simulink model "SWC_FDC_type"  (R2021b)
settings: Solver=FixedStepDiscrete  StartTime=0.0  StopTime=10.0  FixedStep=0.001  RelTol=1e-3
values from neighbouring files (symbols this model uses):
  C_TASK_5MS_S = (	C_TICK_TIME_S      	)    [vcu_local_hdr.m]
  DID_VCUKey = uint16(0x0202)    [vcu_local_hdr.m]
  DID_XWD = uint16(513)    [vcu_local_hdr.m]
  DIDLen_DKCKey = uint16(8)    [vcu_local_hdr.m]
  DIDLen_FoxPiBattSta = uint16(4)    [vcu_local_hdr.m]
  DIDLen_FoxPiBrakeSta = uint16(13)    [vcu_local_hdr.m]
  DIDLen_FoxPiButtonSta = uint16(2)    [vcu_local_hdr.m]
  DIDLen_FoxPiCtrlEnSw = uint16(1)    [vcu_local_hdr.m]
  DIDLen_FoxPiDrivingCtrl = uint16(21)    [vcu_local_hdr.m]
  DIDLen_FoxPiEPSSta = uint16(11)    [vcu_local_hdr.m]
  DIDLen_FoxPiLampCtrl = uint16(6)    [vcu_local_hdr.m]
  DIDLen_FoxPiLampSta = uint16(2)    [vcu_local_hdr.m]
  DIDLen_FoxPiMotionSta = uint16(13)    [vcu_local_hdr.m]
  DIDLen_FoxPiMotorSta = uint16(11)    [vcu_local_hdr.m]
  DIDLen_FoxPiPedalPos = uint16(3)    [vcu_local_hdr.m]
  DIDLen_FoxPiPTGUSSSw = uint16(1)    [vcu_local_hdr.m]
  DIDLen_FoxPiShifterAllow = uint16(3)    [vcu_local_hdr.m]
  DIDLen_FoxPiSwSta = uint16(2)    [vcu_local_hdr.m]
  DIDLen_FoxPiTPMSSta = uint16(13)    [vcu_local_hdr.m]
  DIDLen_FoxPiUSSDist = uint16(20)    [vcu_local_hdr.m]
  DIDLen_FoxPiUSSFaultSta = uint16(2)    [vcu_local_hdr.m]
  DIDLen_FoxPiWheelSpd = uint16(16)    [vcu_local_hdr.m]
  DIDNum_DKCKey = uint16(0x0202)    [vcu_local_hdr.m]
  DIDNum_FoxPiBattSta = uint16(0x100D)    [vcu_local_hdr.m]
  DIDNum_FoxPiBrakeSta = uint16(0x1003)    [vcu_local_hdr.m]
  DIDNum_FoxPiButtonSta = uint16(0x1006)    [vcu_local_hdr.m]
  DIDNum_FoxPiCtrlEnSw = uint16(0x1012)    [vcu_local_hdr.m]
  DIDNum_FoxPiDrivingCtrl = uint16(0x1001)    [vcu_local_hdr.m]
  DIDNum_FoxPiEPSSta = uint16(0x1005)    [vcu_local_hdr.m]
  DIDNum_FoxPiLampCtrl = uint16(0x100C)    [vcu_local_hdr.m]
  DIDNum_FoxPiLampSta = uint16(0x100B)    [vcu_local_hdr.m]
  DIDNum_FoxPiMotionSta = uint16(0x1002)    [vcu_local_hdr.m]
  DIDNum_FoxPiMotorSta = uint16(0x1010)    [vcu_local_hdr.m]
  DIDNum_FoxPiPedalPos = uint16(0x100F)    [vcu_local_hdr.m]
  DIDNum_FoxPiPTGUSSSw = uint16(0x1009)    [vcu_local_hdr.m]
  DIDNum_FoxPiShifterAllow = uint16(0x1011)    [vcu_local_hdr.m]
  DIDNum_FoxPiSwSta = uint16(0x100A)    [vcu_local_hdr.m]
  DIDNum_FoxPiTPMSSta = uint16(0x100E)    [vcu_local_hdr.m]
  DIDNum_FoxPiUSSDist = uint16(0x1007)    [vcu_local_hdr.m]
  DIDNum_FoxPiUSSFaultSta = uint16(0x1008)    [vcu_local_hdr.m]
  DIDNum_FoxPiWheelSpd = uint16(0x1004)    [vcu_local_hdr.m]
  DIDVCUKeyLength = uint16(8)    [vcu_local_hdr.m]
  DTC_10020B = Simulink.Parameter    [DTC_Constant_Definition.m]
  DTC_10020C = Simulink.Parameter    [DTC_Constant_Definition.m]
  DTC_10020D = Simulink.Parameter    [DTC_Constant_Definition.m]
  DTC_10020E = Simulink.Parameter    [DTC_Constant_Definition.m]
  DTC_100210 = Simulink.Parameter    [DTC_Constant_Definition.m]
  DTC_100211 = Simulink.Parameter    [DTC_Constant_Definition.m]
  DTC_100212 = Simulink.Parameter    [DTC_Constant_Definition.m]
  DTC_100213 = Simulink.Parameter    [DTC_Constant_Definition.m]
  DTC_100214 = Simulink.Parameter    [DTC_Constant_Definition.m]
  DTC_100215 = Simulink.Parameter    [DTC_Constant_Definition.m]
  DTC_100216 = Simulink.Parameter    [DTC_Constant_Definition.m]
  DTC_100217 = Simulink.Parameter    [DTC_Constant_Definition.m]
  DTC_100218 = Simulink.Parameter    [DTC_Constant_Definition.m]
  DTC_100219 = Simulink.Parameter    [DTC_Constant_Definition.m]
  DTC_10021A = Simulink.Parameter    [DTC_Constant_Definition.m]
  DTC_10021B = Simulink.Parameter    [DTC_Constant_Definition.m]
  DTC_10021C = Simulink.Parameter    [DTC_Constant_Definition.m]
  DTC_10021D = Simulink.Parameter    [DTC_Constant_Definition.m]
  DTC_10021E = Simulink.Parameter    [DTC_Constant_Definition.m]
  DTC_100220 = Simulink.Parameter    [DTC_Constant_Definition.m]
  DTC_100221 = Simulink.Parameter    [DTC_Constant_Definition.m]
  DTC_100223 = Simulink.Parameter    [DTC_Constant_Definition.m]
  DTC_100224 = Simulink.Parameter    [DTC_Constant_Definition.m]
  DTC_100225 = Simulink.Parameter    [DTC_Constant_Definition.m]
  DTC_100226 = Simulink.Parameter    [DTC_Constant_Definition.m]
  DTC_100227 = Simulink.Parameter    [DTC_Constant_Definition.m]
  DTC_100242 = Simulink.Parameter    [DTC_Constant_Definition.m]
  DTC_100243 = Simulink.Parameter    [DTC_Constant_Definition.m]
  DTC_100244 = Simulink.Parameter    [DTC_Constant_Definition.m]
  DTC_100247 = Simulink.Parameter    [DTC_Constant_Definition.m]
  DTC_100248 = Simulink.Parameter    [DTC_Constant_Definition.m]
  DTC_100249 = Simulink.Parameter    [DTC_Constant_Definition.m]
  DTC_100250 = Simulink.Parameter    [DTC_Constant_Definition.m]
  DTC_100251 = Simulink.Parameter    [DTC_Constant_Definition.m]
  DTC_100252 = Simulink.Parameter    [DTC_Constant_Definition.m]
  DTC_100A10 = Simulink.Parameter    [DTC_Constant_Definition.m]
  DTC_100A12 = Simulink.Parameter    [DTC_Constant_Definition.m]
  DTC_100A16 = Simulink.Parameter    [DTC_Constant_Definition.m]
  DTC_100A17 = Simulink.Parameter    [DTC_Constant_Definition.m]
  DTC_100A18 = Simulink.Parameter    [DTC_Constant_Definition.m]
  DTC_100A19 = Simulink.Parameter    [DTC_Constant_Definition.m]
  DTC_500B01 = Simulink.Parameter    [DTC_Constant_Definition.m]
  DTC_500B02 = Simulink.Parameter    [DTC_Constant_Definition.m]
  DTC_500B03 = Simulink.Parameter    [DTC_Constant_Definition.m]
  DTC_500B04 = Simulink.Parameter    [DTC_Constant_Definition.m]
  DTC_500B05 = Simulink.Parameter    [DTC_Constant_Definition.m]
  DTC_500B06 = Simulink.Parameter    [DTC_Constant_Definition.m]
  DTC_500B07 = Simulink.Parameter    [DTC_Constant_Definition.m]
  DTC_500B08 = Simulink.Parameter    [DTC_Constant_Definition.m]
  DTC_500B09 = Simulink.Parameter    [DTC_Constant_Definition.m]
  DTC_500B0A = Simulink.Parameter    [DTC_Constant_Definition.m]
  DTC_500B0B = Simulink.Parameter    [DTC_Constant_Definition.m]
  DTC_500B0C = Simulink.Parameter    [DTC_Constant_Definition.m]
  DTC_500B0D = Simulink.Parameter    [DTC_Constant_Definition.m]
  DTC_500B0E = Simulink.Parameter    [DTC_Constant_Definition.m]
  DTC_500B0F = Simulink.Parameter    [DTC_Constant_Definition.m]
  DTC_500B10 = Simulink.Parameter    [DTC_Constant_Definition.m]
  DTC_90021F = Simulink.Parameter    [DTC_Constant_Definition.m]
  DTC_90022F = Simulink.Parameter    [DTC_Constant_Definition.m]
  DTC_900253 = Simulink.Parameter    [DTC_Constant_Definition.m]
  DTC_900254 = Simulink.Parameter    [DTC_Constant_Definition.m]
  DTC_900301 = Simulink.Parameter    [DTC_Constant_Definition.m]
  DTC_900302 = Simulink.Parameter    [DTC_Constant_Definition.m]
  DTC_900303 = Simulink.Parameter    [DTC_Constant_Definition.m]
  DTC_900304 = Simulink.Parameter    [DTC_Constant_Definition.m]
  DTC_900305 = Simulink.Parameter    [DTC_Constant_Definition.m]
  DTC_900909 = Simulink.Parameter    [DTC_Constant_Definition.m]
  DTC_90090A = Simulink.Parameter    [DTC_Constant_Definition.m]
  DTC_90090B = Simulink.Parameter    [DTC_Constant_Definition.m]
  DTC_90090C = Simulink.Parameter    [DTC_Constant_Definition.m]
  DTC_90090D = Simulink.Parameter    [DTC_Constant_Definition.m]
  DTC_90090E = Simulink.Parameter    [DTC_Constant_Definition.m]
  DTC_90090F = Simulink.Parameter    [DTC_Constant_Definition.m]
  DTC_900910 = Simulink.Parameter    [DTC_Constant_Definition.m]
  DTC_900911 = Simulink.Parameter    [DTC_Constant_Definition.m]
  DTC_900912 = Simulink.Parameter    [DTC_Constant_Definition.m]
  DTC_900913 = Simulink.Parameter    [DTC_Constant_Definition.m]
  DTC_900914 = Simulink.Parameter    [DTC_Constant_Definition.m]
  ... (+54 more)
undefined symbols (not defined in the file or in its folder): f32_ApsOutVehSpdSig, KHAL_CANBusOffDebounce_cnt, KHAL_CANBusOffDebounce_s, KHAL_DKCDecryptEnable_flg_ovrdflg, KHAL_DKCDecryptEnable_flg_ovrdval, KHAL_RandomNumberY1_enum, KHAL_RandomNumberY2_enum, KHAL_RandomNumberY_ovrdflg, KHAL_TPMSRESBUTT_flg_ovrdflg, KHAL_TPMSRESBUTT_flg_ovrdval, KINP_ReadVinCode_flg, P_boolean, R_DIDWriteCDD_CSOP_DIDSet_DKCKey, R_DIDWriteCDD_CSOP_DIDSet_FoxPiBattSta, R_DIDWriteCDD_CSOP_DIDSet_FoxPiBrakeSta, R_DIDWriteCDD_CSOP_DIDSet_FoxPiButtonSta, R_DIDWriteCDD_CSOP_DIDSet_FoxPiCtrlEnSw, R_DIDWriteCDD_CSOP_DIDSet_FoxPiDrivingCtrl, R_DIDWriteCDD_CSOP_DIDSet_FoxPiEPSSta, R_DIDWriteCDD_CSOP_DIDSet_FoxPiLampCtrl, R_DIDWriteCDD_CSOP_DIDSet_FoxPiLampSta, R_DIDWriteCDD_CSOP_DIDSet_FoxPiMotionSta, R_DIDWriteCDD_CSOP_DIDSet_FoxPiMotorSta, R_DIDWriteCDD_CSOP_DIDSet_FoxPiPedalPos, R_DIDWriteCDD_CSOP_DIDSet_FoxPiPTGUSSSw, R_DIDWriteCDD_CSOP_DIDSet_FoxPiShifterAllow, R_DIDWriteCDD_CSOP_DIDSet_FoxPiSwSta, R_DIDWriteCDD_CSOP_DIDSet_FoxPiTPMSSta, R_DIDWriteCDD_CSOP_DIDSet_FoxPiUSSDist, R_DIDWriteCDD_CSOP_DIDSet_FoxPiUSSFaultSta, R_DIDWriteCDD_CSOP_DIDSet_FoxPiWheelSpd, R_E2E_CAN3_VCU1_CSOP_Write_CAN3_VCU1, R_E2E_CAN3_VCU1_toNIDEC_CSOP_Write_CAN3_VCU1_toNIDEC, R_E2E_CAN4_VCU1_CSOP_Write_CAN4_VCU1, R_FDCCDD_Inner_CSOP_FDC_AppCallSleep, R_HALIN_IMU_CSOP_IMUSetSta, R_HALINCDD_CSOP_PAS_Handler, R_HALINCDD_CSOP_ResetPedalZeroPosDone, R_HALINCDD_CSOP_TPMSSensorIDRegSetResults, R_HALINCDD_CSOP_UDS_Main, R_HALOUT_APS_CSOP_ApsOutput, R_HALOUTCDD_CSOP_AppNmStateReq, R_HALOUTCDD_CSOP_IVIReset, R_HALOUTCDD_CSOP_SetAcoreRebootCmdACK, R_HALOUTCDD_CSOP_SetSysPwrStat ... (+80)
libraries: FVT_lib x447, simulink x289, hcu_lib x19, hdlsllib x9, app x1, halin x1, halout x1, matrix_library x1, inp x1, outp x1
(part 8 of 15)

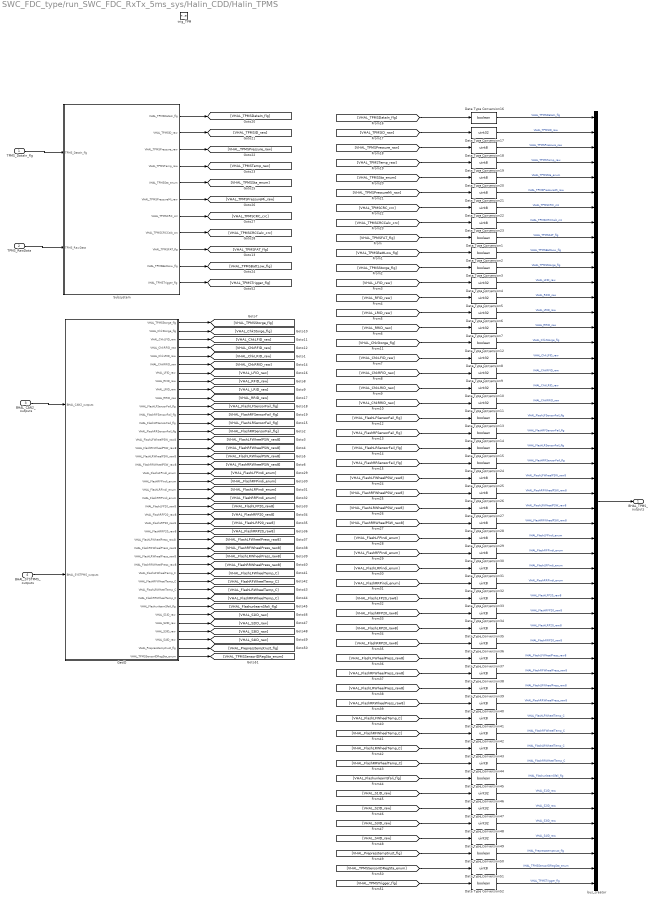
== system SWC_FDC_type/run_SWC_FDC_RxTx_5ms_sys/Halin_CDD/Halin_TPMS ==
  TPMS_DataIn_flg : Inport
  TPMS_RawData : Inport  Port=2
  BHAL_CAN2_outputs : Inport  Port=3
  BHAL_SYSTPMS_outputs : Inport  Port=4
  trig_TPM : TriggerPort  TriggerType=function-call  VariantControl=(inherit)
  Data Type Conversion{1..3,12..16,24,45,50,52} (12 alike) : DataTypeConversion  OutDataTypeStr=boolean
  Data Type Conversion{4..11,17,46..49} (13 alike) : DataTypeConversion  OutDataTypeStr=uint32
  Data Type Conversion{18..23,25..44,51} (27 alike) : DataTypeConversion  OutDataTypeStr=uint8
  GetID : Subsystem
  Subsystem : Subsystem
  bus_creator : BusCreator  Inputs=52  OutDataTypeStr=Bus: BHAL_TPMS_outputs  NonVirtualBus=on
  BHAL_TPMS_outputs : Outport
  wires:
  Subsystem/8(VHAL_TPMSCRCCalc_crc) -> [VHAL_TPMSCRCCalc_crc]
  Subsystem/7(VHAL_TPMSCRC_crc) -> [VHAL_TPMSCRC_crc]
  Subsystem/1(VHAL_TPMSDataIn_flg) -> [VHAL_TPMSDataIn_flg]
  Subsystem/9(VHAL_TPMSFAT_flg) -> [VHAL_TPMSFAT_flg]
  Subsystem/2(VHAL_TPMSID_raw) -> [VHAL_TPMSID_raw]
  Subsystem/10(VHAL_TPMSBattLow_flg) -> [VHAL_TPMSBattLow_flg]
  Subsystem/4(VHAL_TPMSTemp_raw) -> [VHAL_TPMSTemp_raw]
  Subsystem/5(VHAL_TPMSSta_enum) -> [VHAL_TPMSSta_enum]
  Subsystem/3(VHAL_TPMSPressure_raw) -> [VHAL_TPMSPressure_raw]
  Subsystem/6(VHAL_TPMSPressureMi_raw) -> [VHAL_TPMSPressureMi_raw]
  TPMS_DataIn_flg/1 -> Subsystem/1(TPMS_DataIn_flg)
  TPMS_RawData/1 -> Subsystem/2(TPMS_RawData)
  Data Type Conversion29/1 -> bus_creator/29  "VHAL_FlashLFPindi_enum"
  GetID/20(VHAL_FlashRFPindi_enum) -> [VHAL_FlashRFPindi_enum]
  GetID/32(VHAL_FlashRFWheelTemp_C) -> [VHAL_FlashRFWheelTemp_C]
  Data Type Conversion2/1 -> bus_creator/10  "VHAL_TPMSBattLow_flg"
  BHAL_CAN2_outputs/1 -> GetID/1(BHAL_CAN2_outputs)
  [VHAL_TPMSBattLow_flg] -> Data Type Conversion2/1
  [VHAL_FlashLRPindi_enum] -> Data Type Conversion31/1
  [VHAL_FlashunlearnSfali_flg] -> Data Type Conversion45/1
  [VHAL_FlashLFPindi_enum] -> Data Type Conversion29/1
  Data Type Conversion28/1 -> bus_creator/28  "VHAL_FlashRRWheelPSW_raw8"
  [VHAL_FlashLFP20_raw8] -> Data Type Conversion33/1
  [VHAL_RRID_raw] -> Data Type Conversion7/1
  Data Type Conversion42/1 -> bus_creator/42  "VHAL_FlashRFWheelTemp_C"
  Data Type Conversion27/1 -> bus_creator/27  "VHAL_FlashLRWheelPSW_raw8"
  [VHAL_FlashLFWheelTemp_C] -> Data Type Conversion41/1
  Data Type Conversion26/1 -> bus_creator/26  "VHAL_FlashRFWheelPSW_raw8"
  [VHAL_FlashRRP20_raw8] -> Data Type Conversion36/1
  GetID/16(VHAL_FlashRFWheelPSW_raw8) -> [VHAL_FlashRFWheelPSW_raw8]
  [VHAL_RFID_raw] -> Data Type Conversion5/1
  Data Type Conversion33/1 -> bus_creator/33  "VHAL_FlashLFP20_raw8"
  Data Type Conversion24/1 -> bus_creator/24  "VHAL_FlashRRSensorFail_flg"
  Data Type Conversion44/1 -> bus_creator/44  "VHAL_FlashRRWheelTemp_C"
  Data Type Conversion34/1 -> bus_creator/34  "VHAL_FlashRFP20_raw8"
  Data Type Conversion45/1 -> bus_creator/45  "VHAL_FlashunlearnSfali_flg"
  GetID/9(VHAL_LRID_raw) -> [VHAL_LRID_raw]
  Data Type Conversion41/1 -> bus_creator/41  "VHAL_FlashLFWheelTemp_C"
  GetID/15(VHAL_FlashLFWheelPSW_raw8) -> [VHAL_FlashLFWheelPSW_raw8]
  Data Type Conversion15/1 -> bus_creator/23  "VHAL_FlashLRSensorFail_flg"
  [VHAL_FlashLRWheelPress_raw8] -> Data Type Conversion39/1
  Data Type Conversion14/1 -> bus_creator/22  "VHAL_FlashRFSensorFail_flg"
  GetID/34(VHAL_FlashRRWheelTemp_C) -> [VHAL_FlashRRWheelTemp_C]
  Data Type Conversion13/1 -> bus_creator/21  "VHAL_FlashLFSensorFail_flg"
  Data Type Conversion32/1 -> bus_creator/32  "VHAL_FlashRRPindi_enum"
  Data Type Conversion31/1 -> bus_creator/31  "VHAL_FlashLRPindi_enum"
  Data Type Conversion16/1 -> bus_creator/1  "VHAL_TPMSDataIn_flg"
  GetID/22(VHAL_FlashRRPindi_enum) -> [VHAL_FlashRRPindi_enum]
  [VHAL_FlashRFSensorFail_flg] -> Data Type Conversion14/1
  GetID/18(VHAL_FlashRRWheelPSW_raw8) -> [VHAL_FlashRRWheelPSW_raw8]
  Data Type Conversion43/1 -> bus_creator/43  "VHAL_FlashLRWheelTemp_C"
  Data Type Conversion22/1 -> bus_creator/7  "VHAL_TPMSCRC_crc"
  Data Type Conversion40/1 -> bus_creator/40  "VHAL_FlashRRWheelPress_raw8"
  Data Type Conversion39/1 -> bus_creator/39  "VHAL_FlashLRWheelPress_raw8"
  [VHAL_FlashRRPindi_enum] -> Data Type Conversion32/1
  Data Type Conversion38/1 -> bus_creator/38  "VHAL_FlashRFWheelPress_raw8"
  [VHAL_FlashLRP20_raw8] -> Data Type Conversion35/1
  Data Type Conversion35/1 -> bus_creator/35  "VHAL_FlashLRP20_raw8"
  GetID/14(VHAL_FlashRRSensorFail_flg) -> [VHAL_FlashRRSensorFail_flg]
  Data Type Conversion37/1 -> bus_creator/37  "VHAL_FlashLFWheelPress_raw8"
  Data Type Conversion36/1 -> bus_creator/36  "VHAL_FlashRRP20_raw8"
  [VHAL_FlashRRWheelTemp_C] -> Data Type Conversion44/1
  [VHAL_FlashLFWheelPress_raw8] -> Data Type Conversion37/1
  GetID/33(VHAL_FlashLRWheelTemp_C) -> [VHAL_FlashLRWheelTemp_C]
  GetID/26(VHAL_FlashRRP20_raw8) -> [VHAL_FlashRRP20_raw8]
  [VHAL_TPMSFAT_flg] -> Data Type Conversion1/1
  [VHAL_TPMSSta_enum] -> Data Type Conversion20/1
  GetID/25(VHAL_FlashLRP20_raw8) -> [VHAL_FlashLRP20_raw8]
  [VHAL_FlashRRWheelPress_raw8] -> Data Type Conversion40/1
  [VHAL_FlashRFP20_raw8] -> Data Type Conversion34/1
  [VHAL_LFID_raw] -> Data Type Conversion4/1
  [VHAL_FlashRFWheelPSW_raw8] -> Data Type Conversion26/1
  [VHAL_FlashRFWheelTemp_C] -> Data Type Conversion42/1
  [VHAL_FlashLRWheelTemp_C] -> Data Type Conversion43/1
  [VHAL_TPMSCRCCalc_crc] -> Data Type Conversion23/1
  GetID/31(VHAL_FlashLFWheelTemp_C) -> [VHAL_FlashLFWheelTemp_C]
  [VHAL_FlashRRSensorFail_flg] -> Data Type Conversion24/1
  [VHAL_FlashLFSensorFail_flg] -> Data Type Conversion13/1
  GetID/30(VHAL_FlashRRWheelPress_raw8) -> [VHAL_FlashRRWheelPress_raw8]
  Data Type Conversion3/1 -> bus_creator/11  "VHAL_TPMSStorge_flg"
  GetID/29(VHAL_FlashLRWheelPress_raw8) -> [VHAL_FlashLRWheelPress_raw8]
  GetID/21(VHAL_FlashLRPindi_enum) -> [VHAL_FlashLRPindi_enum]
  GetID/1(VHAL_TPMSStorge_flg) -> [VHAL_TPMSStorge_flg]
  [VHAL_FlashRFPindi_enum] -> Data Type Conversion30/1
  GetID/19(VHAL_FlashLFPindi_enum) -> [VHAL_FlashLFPindi_enum]
  GetID/23(VHAL_FlashLFP20_raw8) -> [VHAL_FlashLFP20_raw8]
  Data Type Conversion6/1 -> bus_creator/14  "VHAL_LRID_raw"
  GetID/6(VHAL_ChkRRID_raw) -> [VHAL_ChkRRID_raw]
  [VHAL_TPMSDataIn_flg] -> Data Type Conversion16/1
  GetID/17(VHAL_FlashLRWheelPSW_raw8) -> [VHAL_FlashLRWheelPSW_raw8]
  [VHAL_FlashRFWheelPress_raw8] -> Data Type Conversion38/1
  Data Type Conversion1/1 -> bus_creator/9  "VHAL_TPMSFAT_flg"
  GetID/3(VHAL_ChkLFID_raw) -> [VHAL_ChkLFID_raw]
  GetID/35(VHAL_FlashunlearnSfali_flg) -> [VHAL_FlashunlearnSfali_flg]
  [VHAL_FlashLFWheelPSW_raw8] -> Data Type Conversion25/1
  GetID/8(VHAL_RFID_raw) -> [VHAL_RFID_raw]
  GetID/10(VHAL_RRID_raw) -> [VHAL_RRID_raw]
  Data Type Conversion12/1 -> bus_creator/16  "VHAL_ChkStorge_flg"
  [VHAL_FlashLRWheelPSW_raw8] -> Data Type Conversion27/1
  GetID/7(VHAL_LFID_raw) -> [VHAL_LFID_raw]
  Data Type Conversion18/1 -> bus_creator/3  "VHAL_TPMSPressure_raw"
  Data Type Conversion9/1 -> bus_creator/18  "VHAL_ChkRFID_raw"
  Data Type Conversion10/1 -> bus_creator/19  "VHAL_ChkLRID_raw"
  GetID/11(VHAL_FlashLFSensorFail_flg) -> [VHAL_FlashLFSensorFail_flg]
  GetID/27(VHAL_FlashLFWheelPress_raw8) -> [VHAL_FlashLFWheelPress_raw8]
  Data Type Conversion11/1 -> bus_creator/20  "VHAL_ChkRRID_raw"
  Data Type Conversion7/1 -> bus_creator/15  "VHAL_RRID_raw"
  GetID/4(VHAL_ChkRFID_raw) -> [VHAL_ChkRFID_raw]
  [VHAL_TPMSID_raw] -> Data Type Conversion17/1
  [VHAL_ChkStorge_flg] -> Data Type Conversion12/1
  GetID/28(VHAL_FlashRFWheelPress_raw8) -> [VHAL_FlashRFWheelPress_raw8]
  Data Type Conversion8/1 -> bus_creator/17  "VHAL_ChkLFID_raw"
  [VHAL_ChkRRID_raw] -> Data Type Conversion11/1
  Data Type Conversion4/1 -> bus_creator/12  "VHAL_LFID_raw"
  [VHAL_ChkLRID_raw] -> Data Type Conversion10/1
  [VHAL_ChkLFID_raw] -> Data Type Conversion8/1
  [VHAL_ChkRFID_raw] -> Data Type Conversion9/1
  Data Type Conversion5/1 -> bus_creator/13  "VHAL_RFID_raw"
  [VHAL_LRID_raw] -> Data Type Conversion6/1
  [VHAL_TPMSStorge_flg] -> Data Type Conversion3/1
  GetID/2(VHAL_ChkStorge_flg) -> [VHAL_ChkStorge_flg]
  [VHAL_TPMSCRC_crc] -> Data Type Conversion22/1
  Data Type Conversion19/1 -> bus_creator/4  "VHAL_TPMSTemp_raw"
  BHAL_SYSTPMS_outputs/1 -> GetID/2(BHAL_SYSTPMS_outputs)
  [VHAL_FlashLRSensorFail_flg] -> Data Type Conversion15/1
  Data Type Conversion17/1 -> bus_creator/2  "VHAL_TPMSID_raw"
  Data Type Conversion23/1 -> bus_creator/8  "VHAL_TPMSCRCCalc_crc"
  Data Type Conversion30/1 -> bus_creator/30  "VHAL_FlashRFPindi_enum"
  Data Type Conversion21/1 -> bus_creator/6  "VHAL_TPMSPressureMi_raw"
  GetID/5(VHAL_ChkLRID_raw) -> [VHAL_ChkLRID_raw]
  [VHAL_TPMSTemp_raw] -> Data Type Conversion19/1
  GetID/13(VHAL_FlashLRSensorFail_flg) -> [VHAL_FlashLRSensorFail_flg]
  [VHAL_TPMSPressure_raw] -> Data Type Conversion18/1
  GetID/24(VHAL_FlashRFP20_raw8) -> [VHAL_FlashRFP20_raw8]
  bus_creator/1 -> BHAL_TPMS_outputs/1
  Data Type Conversion20/1 -> bus_creator/5  "VHAL_TPMSSta_enum"
  Data Type Conversion25/1 -> bus_creator/25  "VHAL_FlashLFWheelPSW_raw8"
  [VHAL_TPMSPressureMi_raw] -> Data Type Conversion21/1
  GetID/12(VHAL_FlashRFSensorFail_flg) -> [VHAL_FlashRFSensorFail_flg]
  [VHAL_FlashRRWheelPSW_raw8] -> Data Type Conversion28/1
  GetID/36(VHAL_S1ID_raw) -> [VHAL_S1ID_raw]
  GetID/37(VHAL_S2ID_raw) -> [VHAL_S2ID_raw]
  GetID/38(VHAL_S3ID_raw) -> [VHAL_S3ID_raw]
  GetID/39(VHAL_S4ID_raw) -> [VHAL_S4ID_raw]
  Data Type Conversion46/1 -> bus_creator/46  "VHAL_S1ID_raw"
  Data Type Conversion49/1 -> bus_creator/49  "VHAL_S4ID_raw"
  Data Type Conversion48/1 -> bus_creator/48  "VHAL_S3ID_raw"
  Data Type Conversion47/1 -> bus_creator/47  "VHAL_S2ID_raw"
  [VHAL_S1ID_raw] -> Data Type Conversion46/1
  [VHAL_S2ID_raw] -> Data Type Conversion47/1
  [VHAL_S3ID_raw] -> Data Type Conversion48/1
  [VHAL_S4ID_raw] -> Data Type Conversion49/1
  GetID/40(VHAL_Prepresstemptrust_flg) -> [VHAL_Prepresstemptrust_flg]
  [VHAL_Prepresstemptrust_flg] -> Data Type Conversion50/1
  Data Type Conversion50/1 -> bus_creator/50  "VHAL_Prepresstemptrust_flg"
  GetID/41(VHAL_TPMSSensorIDRegSta_enum) -> [VHAL_TPMSSensorIDRegSta_enum]
  [VHAL_TPMSSensorIDRegSta_enum] -> Data Type Conversion51/1
  Data Type Conversion51/1 -> bus_creator/51  "VHAL_TPMSSensorIDRegSta_enum"
  Subsystem/11(VHAL_TPMSTrigger_flg) -> [VHAL_TPMSTrigger_flg]
  Data Type Conversion52/1 -> bus_creator/52  "VHAL_TPMSTrigger_flg"
  [VHAL_TPMSTrigger_flg] -> Data Type Conversion52/1

== system SWC_FDC_type/run_SWC_FDC_RxTx_5ms_sys/Halin_CDD/Subsystem ==
  VHAL_ClearDTCcmd_flg : Inport
  Bus Creator : BusCreator  Inputs=1
  Data Type Conversion : DataTypeConversion  OutDataTypeStr=boolean
  BHAL_DDM_outputs : Outport  OutDataTypeStr=Bus: BHAL_DDM_outputs
  wires:
  VHAL_ClearDTCcmd_flg/1 -> Data Type Conversion/1
  Bus Creator/1 -> BHAL_DDM_outputs/1
  Data Type Conversion/1 -> Bus Creator/1  "VHAL_ClearDTCcmd_flg"

== system SWC_FDC_type/run_SWC_FDC_RxTx_5ms_sys/OUTP_AFTER/APM ==
  BOUTP_outputs : Inport  OutDataTypeStr=Bus: BOUTP_outputs
  Bus Selector : BusSelector  OutputSignals=VOUTP_VehSpeed_kph,VOUTP_ShiftGearPosn_enum,VOUTP_FSOffSw_enum,VOUTP_VehSpeedTimeOut_flg,VOUTP_FSOffSwTimeOut_flg,VOUTP_ChrgPlugSta_enum
  Data Type Conversion : DataTypeConversion  OutDataTypeStr=single
  Data Type Conversion{1..5} (5 alike) : DataTypeConversion  OutDataTypeStr=uint8
  ApsOut_GearPosnSig : Outport
  ApsOut_SendChrgPlugStaSig : Outport  Port=2
  ApsOut_SetFrSensorOnCmd : Outport  Port=3
  ApsOut_SetFrSensorSwTOCmd : Outport  Port=4
  ApsOut_SetVehSpdTOCmd : Outport  Port=5
  ApsOut_VehSpdSig : Outport  Port=6
  wires:
  BOUTP_outputs/1 -> [BOUTP_outputs]
  [BOUTP_outputs] -> Bus Selector/1
  Bus Selector/1 -> Data Type Conversion/1  "<VOUTP_VehSpeed_kph>"
  Bus Selector/2 -> Data Type Conversion1/1  "<VOUTP_ShiftGearPosn_enum>"
  Bus Selector/3 -> Data Type Conversion2/1  "<VOUTP_FSOffSw_enum>"
  Bus Selector/4 -> Data Type Conversion3/1  "<VOUTP_VehSpeedTimeOut_flg>"
  Bus Selector/5 -> Data Type Conversion4/1  "<VOUTP_FSOffSwTimeOut_flg>"
  Data Type Conversion1/1 -> ApsOut_GearPosnSig/1
  Data Type Conversion2/1 -> ApsOut_SetFrSensorOnCmd/1
  Data Type Conversion4/1 -> ApsOut_SetFrSensorSwTOCmd/1
  Data Type Conversion5/1 -> ApsOut_SendChrgPlugStaSig/1
  Bus Selector/6 -> Data Type Conversion5/1  "<VOUTP_ChrgPlugSta_enum>"
  Data Type Conversion/1 -> ApsOut_VehSpdSig/1
  Data Type Conversion3/1 -> ApsOut_SetVehSpdTOCmd/1
